simulink model "legolab"  (R2023a)
settings: Solver=FixedStepAuto  StartTime=0.0  StopTime=10.0  RelTol=1e-3  EnableMultiTasking=on
libraries: legoev3lib x11
settings Model: ExtModeTrigDuration=2  Creator=eriknymobohne  LastModifiedBy=eriknymobohne
settings SolverCC: PositivePriorityOrder=on
settings OptimizationCC: EnhancedBackFolding=on  PassReuseOutputArgsAs=Individual arguments  ZeroExternalMemoryAtStartup=off  ZeroInternalMemoryAtStartup=off  MaxStackSize=64  OptimizeBlockOrder=speed  DifferentSizesBufferReuse=on  OptimizationCustomize=off  EfficientTunableParamExpr=on
settings DebuggingCC: ParameterTunabilityLossMsg=error
settings HardwareCC: ProdBitPerPointer=32  ProdBitPerSizeT=32  ProdBitPerPtrDiffT=32  ProdLargestAtomicInteger=Long  ProdWordSize=32  ProdHWDeviceType=ARM Compatible->ARM 9  UseEmbeddedCoderFeatures=off  UseSimulinkCoderFeatures=off
settings SFSimCC: MATLABDynamicMemAlloc=off
settings RTWCC: Description=Embedded Coder  SystemTargetFile=ert.tlc  HardwareBoard=LEGO MINDSTORMS EV3  TLCOptions="-aInlineSetEventsForThisBaseRateFcn=TLC_FALSE -aSuppressMultiTaskScheduler=TLC_FALSE  -aRateBasedStepFcn=0"  TemplateMakefile=ert_default_tmf  Toolchain=Sourcery G++ Lite v2009q3
settings CodeAppCC: ForceParamTrailComments=on  IgnoreCustomStorageClasses=off  OperatorAnnotations=on  SimulinkDataObjDesc=on  SFDataObjDesc=on  InsertBlockDesc=on
settings ERTTargetCC: SupportContinuousTime=on  SupportNonInlinedSFcns=on  SupportVariableSizeSignals=on  ExtModeTransport=2  ExtModeStaticAlloc=on  ExtModeMexFile=ext_xcp  ExtModeIntrfLevel=Level2 - Open

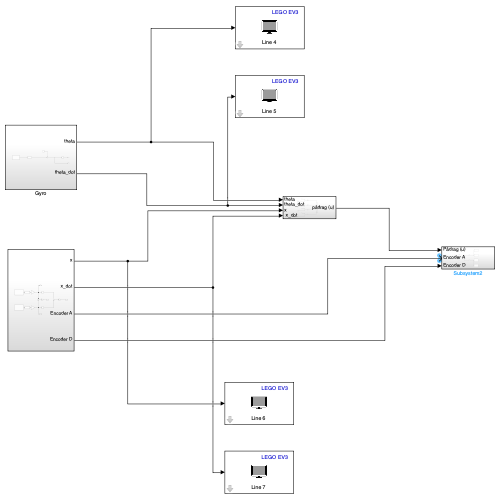
[thumbnail: Simulink's stored preview of the top-level diagram]
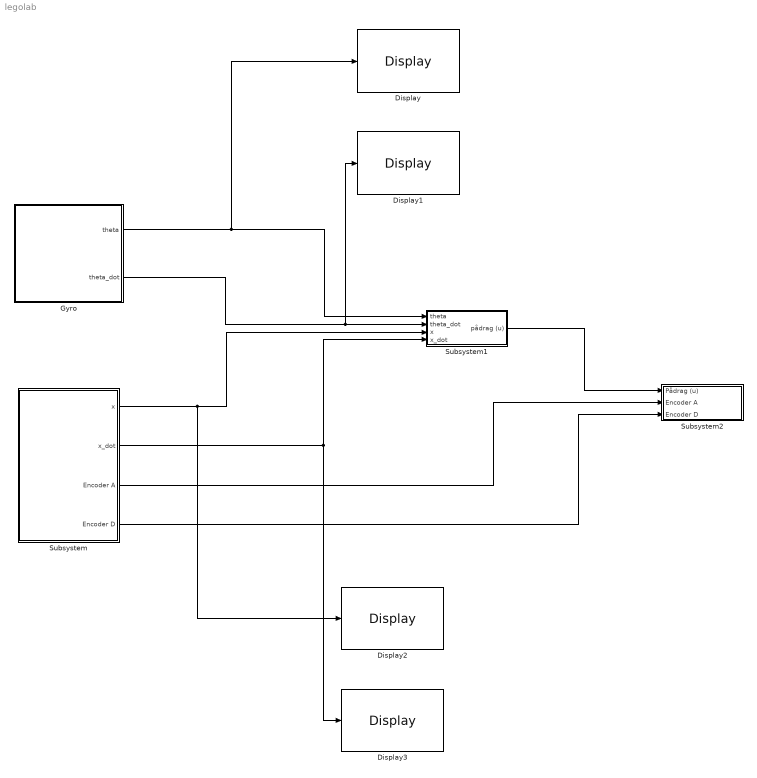
== system legolab ==
  Display : legoev3lib/Display  slcdStr=t  slcdLine=4  slcdFormat=Decimal
  Display1 : legoev3lib/Display  slcdStr=t_dot  slcdLine=5  slcdFormat=Decimal
  Display2 : legoev3lib/Display  slcdStr=x  slcdLine=6  slcdFormat=Decimal
  Display3 : legoev3lib/Display  slcdStr=x_dot  slcdLine=7  slcdFormat=Decimal
  Gyro : Subsystem
  Subsystem : Subsystem
  Subsystem1 : Subsystem
  Subsystem2 : Subsystem
  wires:
  Gyro/1(theta) -> Display/1, Subsystem1/1(theta)
  Gyro/2(theta_dot) -> Display1/1, Subsystem1/2(theta_dot)
  Subsystem/1(x) -> Display2/1, Subsystem1/3(x)
  Subsystem/2(x_dot) -> Display3/1, Subsystem1/4(" x_dot")
  Subsystem/3(Encoder A) -> Subsystem2/2(Encoder A)
  Subsystem/4(Encoder D) -> Subsystem2/3(Encoder D)
  Subsystem1/1(pådrag (u)) -> Subsystem2/1(Pådrag (u))

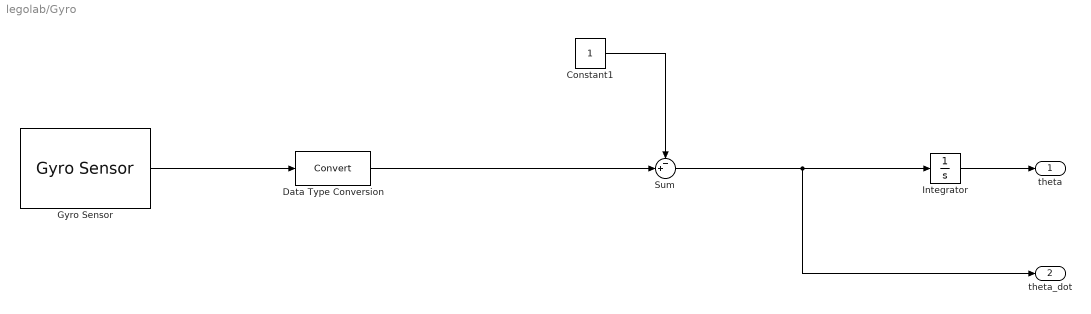
== system legolab/Gyro ==
  Constant1 : Constant
  Data Type Conversion : DataTypeConversion  SaturateOnIntegerOverflow=off  RndMeth=Floor
  Gyro Sensor : legoev3lib/Gyro Sensor  portNumber=2  sampleTime=0.01
  Integrator : Integrator
  Sum : Sum  Inputs=-+|
  theta : Outport
  theta_dot : Outport  Port=2
  wires:
  Gyro Sensor/1 -> Data Type Conversion/1
  Data Type Conversion/1 -> Sum/2
  Integrator/1 -> theta/1
  Constant1/1 -> Sum/1
  Sum/1 -> theta_dot/1, Integrator/1

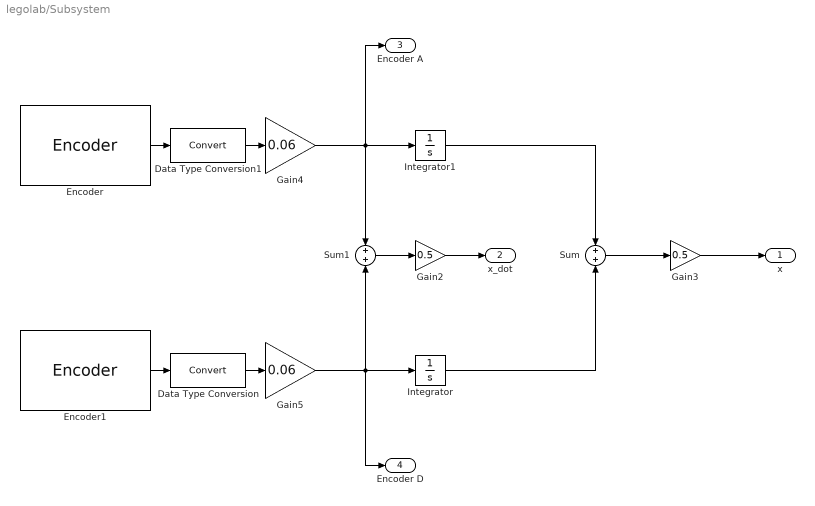
== system legolab/Subsystem ==
  Data Type Conversion : DataTypeConversion  SaturateOnIntegerOverflow=off  RndMeth=Floor
  Data Type Conversion1 : DataTypeConversion  SaturateOnIntegerOverflow=off  RndMeth=Floor
  Encoder : legoev3lib/Encoder  portNumber=A  opMode=Reset at each sample time  sampleTime=0.01
  Encoder1 : legoev3lib/Encoder  portNumber=D  opMode=Reset at each sample time  sampleTime=0.01
  Gain2 : Gain  Gain=0.5
  Gain3 : Gain  Gain=0.5
  Gain4 : Gain  Gain=0.06
  Gain5 : Gain  Gain=0.06
  Integrator : Integrator
  Integrator1 : Integrator
  Sum : Sum  Inputs=+|+
  Sum1 : Sum  Inputs=+|+
  x : Outport
  x_dot : Outport  Port=2
  Encoder A : Outport  Port=3
  Encoder D : Outport  Port=4
  wires:
  Sum1/1 -> Gain2/1
  Gain2/1 -> x_dot/1
  Integrator1/1 -> Sum/1
  Integrator/1 -> Sum/2
  Sum/1 -> Gain3/1
  Gain3/1 -> x/1
  Encoder1/1 -> Data Type Conversion/1
  Encoder/1 -> Data Type Conversion1/1
  Data Type Conversion1/1 -> Gain4/1
  Data Type Conversion/1 -> Gain5/1
  Gain5/1 -> Sum1/2, Integrator/1, Encoder D/1
  Gain4/1 -> Encoder A/1, Sum1/1, Integrator1/1

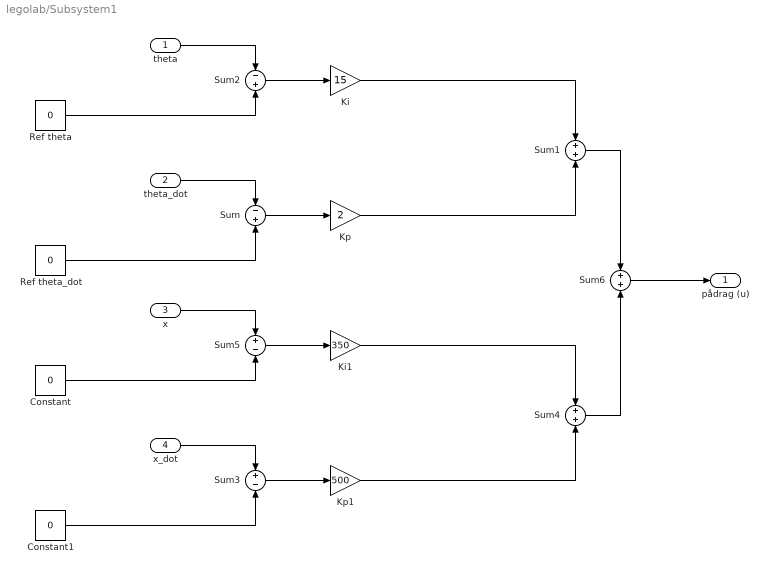
== system legolab/Subsystem1 ==
  theta : Inport
  theta_dot : Inport  Port=2
  x : Inport  Port=3
  " x_dot" : Inport  Port=4
  Constant : Constant  Value=0
  Constant1 : Constant  Value=0
  Ki : Gain  Gain=15
  Ki1 : Gain  Gain=350
  Kp : Gain  Gain=2
  Kp1 : Gain  Gain=500
  Ref theta : Constant  Value=0
  Ref theta_dot : Constant  Value=0
  Sum : Sum  Inputs=-+
  Sum1 : Sum  Inputs=+|+
  Sum2 : Sum  Inputs=-+
  Sum3 : Sum  Inputs=+-
  Sum4 : Sum  Inputs=+|+
  Sum5 : Sum  Inputs=+-
  Sum6 : Sum  Inputs=+|+
  pådrag (u) : Outport
  wires:
  theta_dot/1 -> Sum/1
  Ref theta_dot/1 -> Sum/2
  Sum/1 -> Kp/1
  Ref theta/1 -> Sum2/2
  Sum2/1 -> Ki/1
  theta/1 -> Sum2/1
  Ki/1 -> Sum1/1
  Kp/1 -> Sum1/2
  Sum1/1 -> Sum6/1
  " x_dot"/1 -> Sum3/1
  x/1 -> Sum5/1
  Constant1/1 -> Sum3/2
  Sum5/1 -> Ki1/1
  Ki1/1 -> Sum4/1
  Sum3/1 -> Kp1/1
  Kp1/1 -> Sum4/2
  Sum4/1 -> Sum6/2
  Constant/1 -> Sum5/2
  Sum6/1 -> pådrag (u)/1

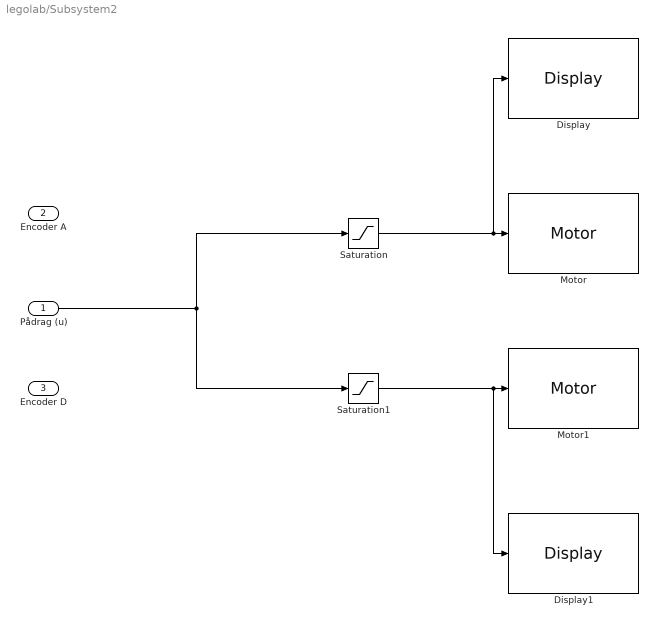
== system legolab/Subsystem2 ==
  Pådrag (u) : Inport
  Encoder A : Inport  Port=2
  Encoder D : Inport  Port=3
  Display : legoev3lib/Display  slcdStr=Motor A  slcdLine=1  slcdFormat=Decimal
  Display1 : legoev3lib/Display  slcdStr=Motor D  slcdLine=1  slcdFormat=Decimal
  Motor : legoev3lib/Motor  sportNumber=A  sstopAction=Brake
  Motor1 : legoev3lib/Motor  sportNumber=D  sstopAction=Brake
  Saturation : Saturate  UpperLimit=100  LowerLimit=-100
  Saturation1 : Saturate  UpperLimit=100  LowerLimit=-100
  wires:
  Saturation/1 -> Display/1, Motor/1
  Saturation1/1 -> Display1/1, Motor1/1
  Pådrag (u)/1 -> Saturation/1, Saturation1/1
